simulink model "verify_heat_exchanger_storage_mdl"  (R2018b)
settings: Solver=ode45  StartTime=0  StopTime=3600  MaxStep=600  RelTol=1e-3  EnableMultiTasking=on
InitFcn:
  | load('DE_TRY2010_13_averageYear')
libraries: carnot x4, carnot_old x1
settings Model: Creator=drhf  LastModifiedBy=P41573
settings DataIOCC: SaveFormat=Array  SignalLoggingSaveFormat=ModelDataLogs
settings OptimizationCC: ExpressionDepthLimit=2147483647  LifeSpan=inf
settings DebuggingCC: UnderspecifiedInitializationDetection=Classic  MergeDetectMultiDrivingBlocksExec=none  SolverPrmCheckMsg=warning  FcnCallInpInsideContextMsg=warning  StateNameClashWarn=warning  SFUnexpectedBacktrackingDiag=warning  SFNoUnconditionalDefaultTransitionDiag=warning  SFExecutionAtInitializationDiag=none
settings HardwareCC: ProdBitPerPointer=32  ProdBitPerSizeT=32  ProdBitPerPtrDiffT=32  ProdLargestAtomicFloat=None  ProdIntDivRoundTo=Undefined  ProdEndianess=Unspecified  ProdWordSize=32  ProdHWDeviceType=32-bit Generic
settings ModelReferenceCC: PropagateSignalLabelsOutOfModel=off
settings SFSimCC: SimUseLocalCustomCode=off
settings RTWCC: RTWUseLocalCustomCode=off
settings CodeAppCC: StateflowObjectComments=on
settings GRTTargetCC: TargetLangStandard=C89/C90 (ANSI)  GeneratePreprocessorConditionals=Disable all  CombineOutputUpdateFcns=off  GRTInterface=on
settings ConfigComp: CovMetricSettings=dw  CovHtmlReporting=on  CovSaveCumulativeToWorkspaceVar=on  CovSaveSingleToWorkspaceVar=on  CovExternalEMLEnable=off

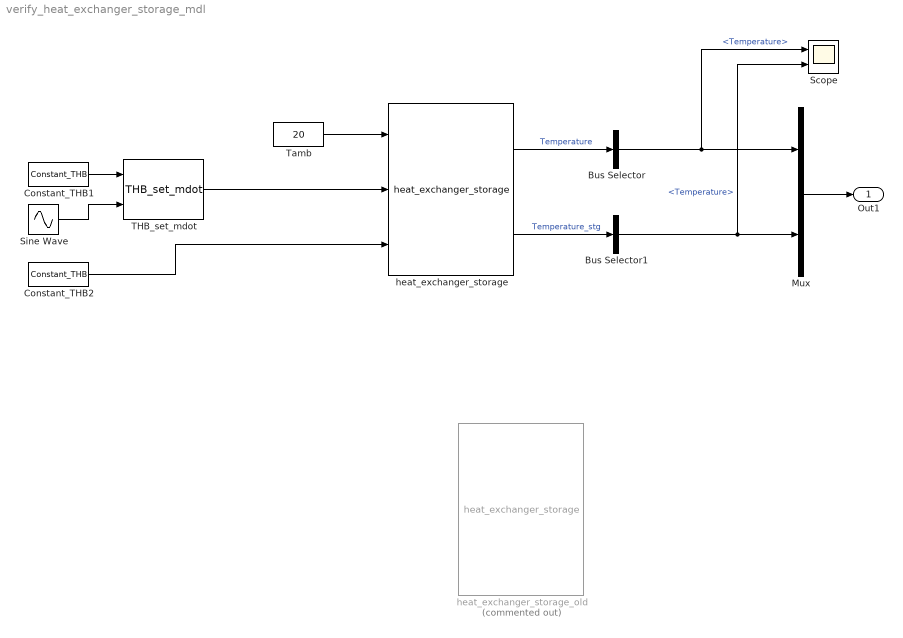
== system verify_heat_exchanger_storage_mdl ==
  Bus Selector : BusSelector  OutputSignals=Temperature
  Bus Selector1 : BusSelector  OutputSignals=Temperature
  Constant_THB1 : carnot/Source/Simple/Constant_THB  t=40  mdot=50/3600  p=1e5  mID=No Pressure Drop  fluid=Water  mix=0  mix2=0  mix3=0  dia=0.02  hgt=0
  Constant_THB2 : carnot/Source/Simple/Constant_THB  t=10  mdot=500/3600  p=1e5  mID=No Pressure Drop  fluid=Water  mix=0  mix2=0  mix3=0  dia=0.02  hgt=0
  Mux : Mux  Inputs=2
  Scope : Scope  NumInputPorts=2
  Sine Wave : Sin  Amplitude=500/3600  Bias=400/3600  Frequency=2*pi/3600  SampleTime=0
  THB_set_mdot : carnot/Source/Simple/THB_set_mdot
  Tamb : Constant  Value=20
  heat_exchanger_storage : carnot/Storage/Thermal/detailed_storage_models/heat_exchanger_storage  v=[0.002 0.0005]  loss=0.1  uh=[500 1]  uc=[500 1]  uw=[300 1]  mat=aluminium  m=[3 0.1]  t0=20  dph=[200 100 1]  dpc=[20 10 0.5]  n=1
  "heat_exchanger_storage_old " : carnot_old/Storage/Thermal/details/heat_exchanger_storage  Commented=on  v=[0.002 0.0005]  loss=0.1  uh=[500 1]  uc=[500 1]  uw=[300 1]  mat=aluminium  m=[3 0.1]  t0=20  dph=[200 100 1]  dpc=[20 10 0.5]  n=1
  Out1 : Outport
  wires:
  Mux/1 -> Out1/1
  Tamb/1 -> heat_exchanger_storage/1
  Constant_THB1/1 -> THB_set_mdot/1
  Sine Wave/1 -> THB_set_mdot/2
  THB_set_mdot/1 -> heat_exchanger_storage/2
  Constant_THB2/1 -> heat_exchanger_storage/3
  heat_exchanger_storage/1 -> Bus Selector/1  "Temperature"
  Bus Selector/1 -> Mux/1, Scope/1  "<Temperature>"
  heat_exchanger_storage/2 -> Bus Selector1/1  "Temperature_stg"
  Bus Selector1/1 -> Mux/2, Scope/2  "<Temperature>"
